simulink model "block_manipulator"  (R2022b)
settings: Solver=ode15s  StartTime=0.0  StopTime=100  FixedStep=0.1  MaxStep=0.01  RelTol=1e-3
values from neighbouring files (symbols this model uses):
  endx = 2    [EnvironmentData.mat]    (also in Practice data.mat = 15)
  endy = 8    [EnvironmentData.mat]    (also in Practice data.mat = 14)
  floorl = 20    [EnvironmentData.mat]    (also in GUIWithNavigation.m; Practice data.mat; RunModel.m)
  floorw = 20    [EnvironmentData.mat]    (also in GUIWithNavigation.m; Practice data.mat; RunModel.m)
  startx = 2    [EnvironmentData.mat]    (also in Practice data.mat)
  starty = 5    [EnvironmentData.mat]    (also in Practice data.mat = 2)
  tar1Len = 3    [EnvironmentData.mat]    (also in GUIWithNavigation.m = length(target1); Practice data.mat = 13; RunModel.m = length(target1))
  target = [2 2.0338184971 1.6 1.6 3.01984057374 1.90928224166 1.77767907717 1.7 5 3.2795509411 2 2 ... (16 elements, 8x2)]    [EnvironmentData.mat]    (also in GUIWithNavigation.m = cat(1,target1,target2); Practice data.mat = [2 3.44057581018 5.07942513831 5.42542290116 7.21306818311 8; RunModel.m = cat(1,target1,target2))
  target1 = [pthObj.States(:,1),pthObj.States(:,2)]    [GUIWithNavigation.m]    (also in RunModel.m)
  target2 = [pthObj.States(:,1),pthObj.States(:,2)]    [GUIWithNavigation.m]    (also in RunModel.m)
undefined symbols (not defined in the file or in its folder): closeFingers, grabObjectAngles, grabObjectAngles2, holdFingers, homeAngles, inverseKinematicWeights, openFingers, readyAngles, X, Y, Z
libraries: sm_lib x199, nesl_utility x57, fl_lib x11, fl_ps_legacy_lib x9, slpidlib x6, robotmaniplib x4
(part 6 of 6)

== system block_manipulator/Manipulator1/j2s6s300_link_finger_3 ==
  Inertia : sm_lib/Body Elements/Inertia  InertiaType=Custom  Mass=0.01  MassUnits=kg  CenterOfMass=[0, 0, 0]  CenterOfMassUnits=m  MomentsOfInertia=[7.8999684e-07, 7.8999684e-07, 8e-08]  MomentsOfInertiaUnits=kg*m^2  ProductsOfInertia=[0, 0, 0]  ProductsOfInertiaUnits=kg*m^2  GraphicType=None  MarkerShape=Inertia  MarkerSize=20  GraphicVisPropType=SimpleVisualProperties  GraphicDiffuseColor=[0.5 0.5 0.5]  GraphicSpecularColor=[0.5 0.5 0.5 1.0]  GraphicAmbientColor=[0.15 0.15 0.15 1.0]  GraphicEmissiveColor=[0.0 0.0 0.0 1.0]  GraphicShininess=75  GraphicOpacity=1.0
  InertiaOriginTransform : sm_lib/Frames and Transforms/Rigid Transform  TranslationMethod=Cartesian  TranslationStandardOffset=0  TranslationLengthUnit=m  TranslationStandardAxis=+Z  TranslationCartesianOffset=[0.022, 0, 0]  TranslationROffset=0  TranslationROffsetUnits=m  TranslationZOffset=0  TranslationZOffsetUnits=m  TranslationThetaOffset=0  TranslationThetaOffsetUnits=deg  RotationMethod=RotationSequence  RotationAngleUnits=deg  RotationStandardAxis=+Z  RotationAngle=0.0  RotationArbitraryAxis=[0 0 1]  FollAlignAxisA=+X  BaseAlignAxisA=+Y  FollAlignAxisB=+Y  BaseAlignAxisB=+Z  RotationSequenceAxes=BaseAxes  RotationSequence=XYZ  RotationSequenceAngles=[0, 0, 0]  RotationSequenceAnglesUnits=rad  RotationMatrix=[1 0 0; 0 1 0; 0 0 1]  Quaternion=[1 0 0 0]
  ReferenceFrame : sm_lib/Frames and Transforms/Reference Frame
  Spatial Contact Force : sm_lib/Forces and Torques/Spatial Contact Force  Commented=on  SenseContactBaseRotation=off  SenseContactBaseTranslation=off  CoefficientOfDynamicFriction=0.3  CoefficientOfStaticFriction=0.5  NormalDamping=1e3  NormalDampingUnits=N/(m/s)  SenseContactSignal=off  NormalStiffness=1e6  NormalStiffnessUnits=N/m  FrictionalCriticalVelocity=1e-3  FrictionalCriticalVelocityUnits=m/s  ZeroCrossDetectContactStartAndEnd=off  SenseContactFollowerRotation=off  SenseContactFollowerTranslation=off  FrictionType=SmoothStickSlip  SenseFrictionalForceMagnitude=off  SenseNormalForceMagnitude=off  NormalForceType=SmoothSpringDamper  SenseNormalVelocity=off  SenseSeparationDistance=off  SenseTangentialVelocity=off  NormalTransitionRegionWidth=1e-4  NormalTransitionRegionWidthUnits=m
  Visual : sm_lib/Body Elements/File Solid  ExtGeomFileName=J2N6S300_finger_proximal.STL  UnitType=Custom  ExtGeomFileUnits=m  StepReaderType=HEX  ExportConvexHullGeometry=on  InertiaType=Custom  Mass=0  MassUnits=kg  CenterOfMass=[0, 0, 0]  CenterOfMassUnits=m  MomentsOfInertia=[0, 0, 0]  MomentsOfInertiaUnits=kg*m^2  ProductsOfInertia=[0, 0, 0]  ProductsOfInertiaUnits=kg*m^2  BasedOnType=DensityFromFile  Density=1000  DensityUnits=kg/m^3  DoExposeReferenceFrame=on  SerializedFrames=<Frames/>  GraphicType=FromGeometry  MarkerShape=Sphere  MarkerSize=10  GraphicVisPropType=SimpleVisualProperties  GraphicDiffuseColor=[0.7254901, 0.490196, 0.062745]  GraphicSpecularColor=[0.5 0.5 0.5 1.0]  GraphicAmbientColor=[0.15 0.15 0.15 1.0]  GraphicEmissiveColor=[0.0 0.0 0.0 1.0]  GraphicShininess=75  GraphicOpacity=1
  VisualOriginTransform : sm_lib/Frames and Transforms/Rigid Transform  TranslationMethod=Cartesian  TranslationStandardOffset=0  TranslationLengthUnit=m  TranslationStandardAxis=+Z  TranslationCartesianOffset=[0, 0, 0]  TranslationROffset=0  TranslationROffsetUnits=m  TranslationZOffset=0  TranslationZOffsetUnits=m  TranslationThetaOffset=0  TranslationThetaOffsetUnits=deg  RotationMethod=RotationSequence  RotationAngleUnits=deg  RotationStandardAxis=+Z  RotationAngle=0.0  RotationArbitraryAxis=[0 0 1]  FollAlignAxisA=+X  BaseAlignAxisA=+Y  FollAlignAxisB=+Y  BaseAlignAxisB=+Z  RotationSequenceAxes=BaseAxes  RotationSequence=XYZ  RotationSequenceAngles=[0, 0, 0]  RotationSequenceAnglesUnits=rad  RotationMatrix=[1 0 0; 0 1 0; 0 0 1]  Quaternion=[1 0 0 0]
  j2s6s300_joint_finger_3_AxisInvTransform : sm_lib/Frames and Transforms/Rigid Transform  TranslationMethod=Cartesian  TranslationStandardOffset=0  TranslationLengthUnit=m  TranslationStandardAxis=+Z  TranslationCartesianOffset=[0, 0, 0]  TranslationROffset=0  TranslationROffsetUnits=m  TranslationZOffset=0  TranslationZOffsetUnits=m  TranslationThetaOffset=0  TranslationThetaOffsetUnits=deg  RotationMethod=ArbitraryAxis  RotationAngleUnits=rad  RotationStandardAxis=+Z  RotationAngle=0  RotationArbitraryAxis=[1, 0, 0]  FollAlignAxisA=+X  BaseAlignAxisA=+Y  FollAlignAxisB=+Y  BaseAlignAxisB=+Z  RotationSequenceAxes=FollowerAxes  RotationSequence=XYX  RotationSequenceAngles=[0 0 0]  RotationSequenceAnglesUnits=deg  RotationMatrix=[1 0 0; 0 1 0; 0 0 1]  Quaternion=[1 0 0 0]
  j2s6s300_joint_finger_tip_3_OriginTransform : sm_lib/Frames and Transforms/Rigid Transform  TranslationMethod=Cartesian  TranslationStandardOffset=0  TranslationLengthUnit=m  TranslationStandardAxis=+Z  TranslationCartesianOffset=[0.044, -0.003, 0]  TranslationROffset=0  TranslationROffsetUnits=m  TranslationZOffset=0  TranslationZOffsetUnits=m  TranslationThetaOffset=0  TranslationThetaOffsetUnits=deg  RotationMethod=RotationSequence  RotationAngleUnits=deg  RotationStandardAxis=+Z  RotationAngle=0.0  RotationArbitraryAxis=[0 0 1]  FollAlignAxisA=+X  BaseAlignAxisA=+Y  FollAlignAxisB=+Y  BaseAlignAxisB=+Z  RotationSequenceAxes=BaseAxes  RotationSequence=XYZ  RotationSequenceAngles=[0, 0, 0]  RotationSequenceAnglesUnits=rad  RotationMatrix=[1 0 0; 0 1 0; 0 0 1]  Quaternion=[1 0 0 0]
  F : PMIOPort  Side=Left
  F1 : PMIOPort  Port=2  Side=Right
  Block1 Contact Force : PMIOPort  Port=3  Side=Right
  connections:
  Inertia/RConn1 -- InertiaOriginTransform/RConn1
  InertiaOriginTransform/LConn1 -- j2s6s300_joint_finger_3_AxisInvTransform/LConn1 -- j2s6s300_joint_finger_tip_3_OriginTransform/LConn1 -- VisualOriginTransform/LConn1 -- ReferenceFrame/RConn1
  Visual/RConn1 -- VisualOriginTransform/RConn1
  j2s6s300_joint_finger_3_AxisInvTransform/RConn1 -- F/RConn1
  j2s6s300_joint_finger_tip_3_OriginTransform/RConn1 -- F1/RConn1
  Spatial Contact Force/RConn1 -- Block1 Contact Force/RConn1
  Spatial Contact Force/LConn1 -- Visual/LConn1

== system block_manipulator/Manipulator1/j2s6s300_link_finger_tip_1 ==
  Inertia : sm_lib/Body Elements/Inertia  InertiaType=Custom  Mass=0.01  MassUnits=kg  CenterOfMass=[0, 0, 0]  CenterOfMassUnits=m  MomentsOfInertia=[7.8999684e-07, 7.8999684e-07, 8e-08]  MomentsOfInertiaUnits=kg*m^2  ProductsOfInertia=[0, 0, 0]  ProductsOfInertiaUnits=kg*m^2  GraphicType=None  MarkerShape=Inertia  MarkerSize=20  GraphicVisPropType=SimpleVisualProperties  GraphicDiffuseColor=[0.5 0.5 0.5]  GraphicSpecularColor=[0.5 0.5 0.5 1.0]  GraphicAmbientColor=[0.15 0.15 0.15 1.0]  GraphicEmissiveColor=[0.0 0.0 0.0 1.0]  GraphicShininess=75  GraphicOpacity=1.0
  InertiaOriginTransform : sm_lib/Frames and Transforms/Rigid Transform  TranslationMethod=Cartesian  TranslationStandardOffset=0  TranslationLengthUnit=m  TranslationStandardAxis=+Z  TranslationCartesianOffset=[0.022, 0, 0]  TranslationROffset=0  TranslationROffsetUnits=m  TranslationZOffset=0  TranslationZOffsetUnits=m  TranslationThetaOffset=0  TranslationThetaOffsetUnits=deg  RotationMethod=RotationSequence  RotationAngleUnits=deg  RotationStandardAxis=+Z  RotationAngle=0.0  RotationArbitraryAxis=[0 0 1]  FollAlignAxisA=+X  BaseAlignAxisA=+Y  FollAlignAxisB=+Y  BaseAlignAxisB=+Z  RotationSequenceAxes=BaseAxes  RotationSequence=XYZ  RotationSequenceAngles=[0, 0, 0]  RotationSequenceAnglesUnits=rad  RotationMatrix=[1 0 0; 0 1 0; 0 0 1]  Quaternion=[1 0 0 0]
  ReferenceFrame : sm_lib/Frames and Transforms/Reference Frame
  Spatial Contact Force : sm_lib/Forces and Torques/Spatial Contact Force  Commented=on  SenseContactBaseRotation=off  SenseContactBaseTranslation=off  CoefficientOfDynamicFriction=0.9  CoefficientOfStaticFriction=0.9  NormalDamping=1e3  NormalDampingUnits=N/(m/s)  SenseContactSignal=off  NormalStiffness=1e6  NormalStiffnessUnits=N/m  FrictionalCriticalVelocity=1e-3  FrictionalCriticalVelocityUnits=m/s  ZeroCrossDetectContactStartAndEnd=off  SenseContactFollowerRotation=off  SenseContactFollowerTranslation=off  FrictionType=SmoothStickSlip  SenseFrictionalForceMagnitude=off  SenseNormalForceMagnitude=on  NormalForceType=SmoothSpringDamper  SenseNormalVelocity=off  SenseSeparationDistance=off  SenseTangentialVelocity=off  NormalTransitionRegionWidth=1e-4  NormalTransitionRegionWidthUnits=m
  Visual : sm_lib/Body Elements/File Solid  ExtGeomFileName=J2N6S300_finger_distal.STL  UnitType=Custom  ExtGeomFileUnits=m  StepReaderType=HEX  ExportConvexHullGeometry=on  InertiaType=Custom  Mass=0  MassUnits=kg  CenterOfMass=[0, 0, 0]  CenterOfMassUnits=m  MomentsOfInertia=[0, 0, 0]  MomentsOfInertiaUnits=kg*m^2  ProductsOfInertia=[0, 0, 0]  ProductsOfInertiaUnits=kg*m^2  BasedOnType=DensityFromFile  Density=1000  DensityUnits=kg/m^3  DoExposeReferenceFrame=on  SerializedFrames=<Frames/>  GraphicType=FromGeometry  MarkerShape=Sphere  MarkerSize=10  GraphicVisPropType=SimpleVisualProperties  GraphicDiffuseColor=[0.4156862, 0.0470588, 0.0431372]  GraphicSpecularColor=[0.5 0.5 0.5 1.0]  GraphicAmbientColor=[0.15 0.15 0.15 1.0]  GraphicEmissiveColor=[0.0 0.0 0.0 1.0]  GraphicShininess=75  GraphicOpacity=1
  VisualOriginTransform : sm_lib/Frames and Transforms/Rigid Transform  TranslationMethod=Cartesian  TranslationStandardOffset=0  TranslationLengthUnit=m  TranslationStandardAxis=+Z  TranslationCartesianOffset=[0, 0, 0]  TranslationROffset=0  TranslationROffsetUnits=m  TranslationZOffset=0  TranslationZOffsetUnits=m  TranslationThetaOffset=0  TranslationThetaOffsetUnits=deg  RotationMethod=RotationSequence  RotationAngleUnits=deg  RotationStandardAxis=+Z  RotationAngle=0.0  RotationArbitraryAxis=[0 0 1]  FollAlignAxisA=+X  BaseAlignAxisA=+Y  FollAlignAxisB=+Y  BaseAlignAxisB=+Z  RotationSequenceAxes=BaseAxes  RotationSequence=XYZ  RotationSequenceAngles=[0, 0, 0]  RotationSequenceAnglesUnits=rad  RotationMatrix=[1 0 0; 0 1 0; 0 0 1]  Quaternion=[1 0 0 0]
  F : PMIOPort  Side=Left
  Block1 Contact Force : PMIOPort  Port=2  Side=Right
  F1 : PMIOPort  Port=3  Side=Left
  connections:
  Inertia/RConn1 -- InertiaOriginTransform/RConn1
  InertiaOriginTransform/LConn1 -- ReferenceFrame/RConn1 -- F/RConn1 -- VisualOriginTransform/LConn1
  Visual/RConn1 -- VisualOriginTransform/RConn1
  Visual/LConn1 -- Spatial Contact Force/LConn1
  Spatial Contact Force/RConn1 -- Block1 Contact Force/RConn1
  F1/RConn1 -- Spatial Contact Force/RConn2

== system block_manipulator/Manipulator1/j2s6s300_link_finger_tip_2 ==
  Inertia : sm_lib/Body Elements/Inertia  InertiaType=Custom  Mass=0.01  MassUnits=kg  CenterOfMass=[0, 0, 0]  CenterOfMassUnits=m  MomentsOfInertia=[7.8999684e-07, 7.8999684e-07, 8e-08]  MomentsOfInertiaUnits=kg*m^2  ProductsOfInertia=[0, 0, 0]  ProductsOfInertiaUnits=kg*m^2  GraphicType=None  MarkerShape=Inertia  MarkerSize=20  GraphicVisPropType=SimpleVisualProperties  GraphicDiffuseColor=[0.5 0.5 0.5]  GraphicSpecularColor=[0.5 0.5 0.5 1.0]  GraphicAmbientColor=[0.15 0.15 0.15 1.0]  GraphicEmissiveColor=[0.0 0.0 0.0 1.0]  GraphicShininess=75  GraphicOpacity=1.0
  InertiaOriginTransform : sm_lib/Frames and Transforms/Rigid Transform  TranslationMethod=Cartesian  TranslationStandardOffset=0  TranslationLengthUnit=m  TranslationStandardAxis=+Z  TranslationCartesianOffset=[0.022, 0, 0]  TranslationROffset=0  TranslationROffsetUnits=m  TranslationZOffset=0  TranslationZOffsetUnits=m  TranslationThetaOffset=0  TranslationThetaOffsetUnits=deg  RotationMethod=RotationSequence  RotationAngleUnits=deg  RotationStandardAxis=+Z  RotationAngle=0.0  RotationArbitraryAxis=[0 0 1]  FollAlignAxisA=+X  BaseAlignAxisA=+Y  FollAlignAxisB=+Y  BaseAlignAxisB=+Z  RotationSequenceAxes=BaseAxes  RotationSequence=XYZ  RotationSequenceAngles=[0, 0, 0]  RotationSequenceAnglesUnits=rad  RotationMatrix=[1 0 0; 0 1 0; 0 0 1]  Quaternion=[1 0 0 0]
  ReferenceFrame : sm_lib/Frames and Transforms/Reference Frame
  Spatial Contact Force : sm_lib/Forces and Torques/Spatial Contact Force  Commented=on  SenseContactBaseRotation=off  SenseContactBaseTranslation=off  CoefficientOfDynamicFriction=0.9  CoefficientOfStaticFriction=0.9  NormalDamping=1e3  NormalDampingUnits=N/(m/s)  SenseContactSignal=off  NormalStiffness=1e6  NormalStiffnessUnits=N/m  FrictionalCriticalVelocity=1e-3  FrictionalCriticalVelocityUnits=m/s  ZeroCrossDetectContactStartAndEnd=off  SenseContactFollowerRotation=off  SenseContactFollowerTranslation=off  FrictionType=SmoothStickSlip  SenseFrictionalForceMagnitude=off  SenseNormalForceMagnitude=on  NormalForceType=SmoothSpringDamper  SenseNormalVelocity=off  SenseSeparationDistance=off  SenseTangentialVelocity=off  NormalTransitionRegionWidth=1e-4  NormalTransitionRegionWidthUnits=m
  Visual : sm_lib/Body Elements/File Solid  ExtGeomFileName=J2N6S300_finger_distal.STL  UnitType=Custom  ExtGeomFileUnits=m  StepReaderType=HEX  ExportConvexHullGeometry=on  InertiaType=Custom  Mass=0  MassUnits=kg  CenterOfMass=[0, 0, 0]  CenterOfMassUnits=m  MomentsOfInertia=[0, 0, 0]  MomentsOfInertiaUnits=kg*m^2  ProductsOfInertia=[0, 0, 0]  ProductsOfInertiaUnits=kg*m^2  BasedOnType=DensityFromFile  Density=1000  DensityUnits=kg/m^3  DoExposeReferenceFrame=on  SerializedFrames=<Frames/>  GraphicType=FromGeometry  MarkerShape=Sphere  MarkerSize=10  GraphicVisPropType=SimpleVisualProperties  GraphicDiffuseColor=[0.4156862, 0.0470588, 0.0431372]  GraphicSpecularColor=[0.5 0.5 0.5 1.0]  GraphicAmbientColor=[0.15 0.15 0.15 1.0]  GraphicEmissiveColor=[0.0 0.0 0.0 1.0]  GraphicShininess=75  GraphicOpacity=1
  VisualOriginTransform : sm_lib/Frames and Transforms/Rigid Transform  TranslationMethod=Cartesian  TranslationStandardOffset=0  TranslationLengthUnit=m  TranslationStandardAxis=+Z  TranslationCartesianOffset=[0, 0, 0]  TranslationROffset=0  TranslationROffsetUnits=m  TranslationZOffset=0  TranslationZOffsetUnits=m  TranslationThetaOffset=0  TranslationThetaOffsetUnits=deg  RotationMethod=RotationSequence  RotationAngleUnits=deg  RotationStandardAxis=+Z  RotationAngle=0.0  RotationArbitraryAxis=[0 0 1]  FollAlignAxisA=+X  BaseAlignAxisA=+Y  FollAlignAxisB=+Y  BaseAlignAxisB=+Z  RotationSequenceAxes=BaseAxes  RotationSequence=XYZ  RotationSequenceAngles=[0, 0, 0]  RotationSequenceAnglesUnits=rad  RotationMatrix=[1 0 0; 0 1 0; 0 0 1]  Quaternion=[1 0 0 0]
  F : PMIOPort  Side=Left
  Block1 Contact Force : PMIOPort  Port=2  Side=Right
  F1 : PMIOPort  Port=3  Side=Left
  connections:
  Inertia/RConn1 -- InertiaOriginTransform/RConn1
  InertiaOriginTransform/LConn1 -- ReferenceFrame/RConn1 -- F/RConn1 -- VisualOriginTransform/LConn1
  Visual/RConn1 -- VisualOriginTransform/RConn1
  Visual/LConn1 -- Spatial Contact Force/LConn1
  Block1 Contact Force/RConn1 -- Spatial Contact Force/RConn1
  Spatial Contact Force/RConn2 -- F1/RConn1

== system block_manipulator/Manipulator1/j2s6s300_link_finger_tip_3 ==
  Inertia : sm_lib/Body Elements/Inertia  InertiaType=Custom  Mass=0.01  MassUnits=kg  CenterOfMass=[0, 0, 0]  CenterOfMassUnits=m  MomentsOfInertia=[7.8999684e-07, 7.8999684e-07, 8e-08]  MomentsOfInertiaUnits=kg*m^2  ProductsOfInertia=[0, 0, 0]  ProductsOfInertiaUnits=kg*m^2  GraphicType=None  MarkerShape=Inertia  MarkerSize=20  GraphicVisPropType=SimpleVisualProperties  GraphicDiffuseColor=[0.5 0.5 0.5]  GraphicSpecularColor=[0.5 0.5 0.5 1.0]  GraphicAmbientColor=[0.15 0.15 0.15 1.0]  GraphicEmissiveColor=[0.0 0.0 0.0 1.0]  GraphicShininess=75  GraphicOpacity=1.0
  InertiaOriginTransform : sm_lib/Frames and Transforms/Rigid Transform  TranslationMethod=Cartesian  TranslationStandardOffset=0  TranslationLengthUnit=m  TranslationStandardAxis=+Z  TranslationCartesianOffset=[0.022, 0, 0]  TranslationROffset=0  TranslationROffsetUnits=m  TranslationZOffset=0  TranslationZOffsetUnits=m  TranslationThetaOffset=0  TranslationThetaOffsetUnits=deg  RotationMethod=RotationSequence  RotationAngleUnits=deg  RotationStandardAxis=+Z  RotationAngle=0.0  RotationArbitraryAxis=[0 0 1]  FollAlignAxisA=+X  BaseAlignAxisA=+Y  FollAlignAxisB=+Y  BaseAlignAxisB=+Z  RotationSequenceAxes=BaseAxes  RotationSequence=XYZ  RotationSequenceAngles=[0, 0, 0]  RotationSequenceAnglesUnits=rad  RotationMatrix=[1 0 0; 0 1 0; 0 0 1]  Quaternion=[1 0 0 0]
  ReferenceFrame : sm_lib/Frames and Transforms/Reference Frame
  Spatial Contact Force : sm_lib/Forces and Torques/Spatial Contact Force  Commented=on  SenseContactBaseRotation=off  SenseContactBaseTranslation=off  CoefficientOfDynamicFriction=0.9  CoefficientOfStaticFriction=0.9  NormalDamping=1e3  NormalDampingUnits=N/(m/s)  SenseContactSignal=off  NormalStiffness=1e6  NormalStiffnessUnits=N/m  FrictionalCriticalVelocity=1e-3  FrictionalCriticalVelocityUnits=m/s  ZeroCrossDetectContactStartAndEnd=off  SenseContactFollowerRotation=off  SenseContactFollowerTranslation=off  FrictionType=SmoothStickSlip  SenseFrictionalForceMagnitude=off  SenseNormalForceMagnitude=on  NormalForceType=SmoothSpringDamper  SenseNormalVelocity=off  SenseSeparationDistance=off  SenseTangentialVelocity=off  NormalTransitionRegionWidth=1e-4  NormalTransitionRegionWidthUnits=m
  Visual : sm_lib/Body Elements/File Solid  ExtGeomFileName=J2N6S300_finger_distal.STL  UnitType=Custom  ExtGeomFileUnits=m  StepReaderType=HEX  ExportConvexHullGeometry=on  InertiaType=Custom  Mass=0  MassUnits=kg  CenterOfMass=[0, 0, 0]  CenterOfMassUnits=m  MomentsOfInertia=[0, 0, 0]  MomentsOfInertiaUnits=kg*m^2  ProductsOfInertia=[0, 0, 0]  ProductsOfInertiaUnits=kg*m^2  BasedOnType=DensityFromFile  Density=1000  DensityUnits=kg/m^3  DoExposeReferenceFrame=on  SerializedFrames=<Frames/>  GraphicType=FromGeometry  MarkerShape=Sphere  MarkerSize=10  GraphicVisPropType=SimpleVisualProperties  GraphicDiffuseColor=[0.4156862, 0.0470588, 0.0431372]  GraphicSpecularColor=[0.5 0.5 0.5 1.0]  GraphicAmbientColor=[0.15 0.15 0.15 1.0]  GraphicEmissiveColor=[0.0 0.0 0.0 1.0]  GraphicShininess=75  GraphicOpacity=1
  VisualOriginTransform : sm_lib/Frames and Transforms/Rigid Transform  TranslationMethod=Cartesian  TranslationStandardOffset=0  TranslationLengthUnit=m  TranslationStandardAxis=+Z  TranslationCartesianOffset=[0, 0, 0]  TranslationROffset=0  TranslationROffsetUnits=m  TranslationZOffset=0  TranslationZOffsetUnits=m  TranslationThetaOffset=0  TranslationThetaOffsetUnits=deg  RotationMethod=RotationSequence  RotationAngleUnits=deg  RotationStandardAxis=+Z  RotationAngle=0.0  RotationArbitraryAxis=[0 0 1]  FollAlignAxisA=+X  BaseAlignAxisA=+Y  FollAlignAxisB=+Y  BaseAlignAxisB=+Z  RotationSequenceAxes=BaseAxes  RotationSequence=XYZ  RotationSequenceAngles=[0, 0, 0]  RotationSequenceAnglesUnits=rad  RotationMatrix=[1 0 0; 0 1 0; 0 0 1]  Quaternion=[1 0 0 0]
  F : PMIOPort  Side=Left
  Block1 Contact Force : PMIOPort  Port=2  Side=Right
  F1 : PMIOPort  Port=3  Side=Left
  connections:
  Inertia/RConn1 -- InertiaOriginTransform/RConn1
  InertiaOriginTransform/LConn1 -- ReferenceFrame/RConn1 -- F/RConn1 -- VisualOriginTransform/LConn1
  Visual/RConn1 -- VisualOriginTransform/RConn1
  Visual/LConn1 -- Spatial Contact Force/LConn1
  Block1 Contact Force/RConn1 -- Spatial Contact Force/RConn1
  F1/RConn1 -- Spatial Contact Force/RConn2

== system block_manipulator/Controller/Path follower/If Action Subsystem ==
  In1 : Inport
  Action Port : ActionPort  ActionPortLabel=if(u1 <= 0)
  Out1 : Outport
  wires:
  In1/1 -> Out1/1

== system block_manipulator/Controller/Path follower/If Action Subsystem1 ==
  In1 : Inport
  Action Port : ActionPort  ActionPortLabel=else
  Out1 : Outport
  wires:
  In1/1 -> Out1/1

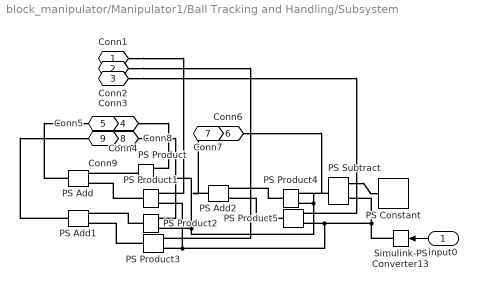
== system block_manipulator/Manipulator1/Ball Tracking and Handling/Subsystem ==
  input0 : Inport
  PS Add : fl_lib/Physical Signals/Functions/PS Add
  PS Add1 : fl_lib/Physical Signals/Functions/PS Add
  PS Add2 : fl_lib/Physical Signals/Functions/PS Add
  PS Constant : fl_lib/Physical Signals/Sources/PS Constant  constant=1
  PS Product{,1..5} (6 alike) : fl_ps_legacy_lib/Legacy Physical Signals/Functions/PS Product
  PS Subtract : fl_lib/Physical Signals/Functions/PS Subtract
  Simulink-PS Converter13 : nesl_utility/Simulink-PS Converter  PhysicalDomain=network_engine_domain  SubClassName=ps_input  LeftPortType=input  RightPortType=output  PseudoPeriodic=off  Frequencies=[]  NoiseDistribution=none  NoiseParameters=[]  Unit=1  AffineConversion=off  FilteringAndDerivatives=provide  SimscapeFilterOrder=1  InputFilterTimeConstant=0.001  UdotUserProvided=0
  Conn1 : PMIOPort  Side=Left
  Conn2 : PMIOPort  Port=2  Side=Left
  Conn3 : PMIOPort  Port=3  Side=Left
  Conn4 : PMIOPort  Port=4  Side=Right
  Conn5 : PMIOPort  Port=5  Side=Left
  Conn6 : PMIOPort  Port=6  Side=Right
  Conn7 : PMIOPort  Port=7  Side=Left
  Conn8 : PMIOPort  Port=8  Side=Right
  Conn9 : PMIOPort  Port=9  Side=Left
  wires:
  input0/1 -> Simulink-PS Converter13/1
  connections:
  PS Product3/RConn1 -- PS Add1/LConn2
  PS Subtract/RConn1 -- PS Product/LConn1 -- PS Product2/LConn1 -- PS Product4/LConn1
  PS Product/RConn1 -- PS Add/LConn1
  PS Product4/RConn1 -- PS Add2/LConn1
  Conn2/RConn1 -- PS Product3/LConn2
  PS Add1/RConn1 -- Conn8/RConn1
  PS Product2/RConn1 -- PS Add1/LConn1
  PS Product5/RConn1 -- PS Add2/LConn2
  PS Subtract/LConn1 -- PS Constant/RConn1
  Simulink-PS Converter13/RConn1 -- PS Product1/LConn1 -- PS Product3/LConn1 -- PS Product5/LConn1 -- PS Subtract/LConn2
  PS Product1/RConn1 -- PS Add/LConn2
  Conn7/RConn1 -- PS Product4/LConn2
  Conn5/RConn1 -- PS Product/LConn2
  Conn9/RConn1 -- PS Product2/LConn2
  PS Add/RConn1 -- Conn4/RConn1
  Conn3/RConn1 -- PS Product5/LConn2
  Conn1/RConn1 -- PS Product1/LConn2
  PS Add2/RConn1 -- Conn6/RConn1

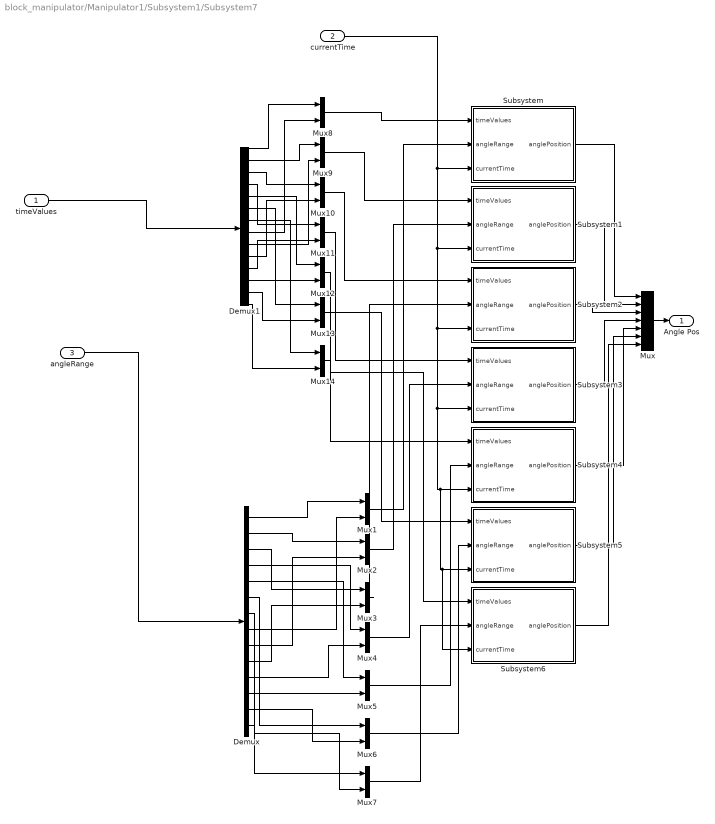
== system block_manipulator/Manipulator1/Subsystem1/Subsystem7 ==
  timeValues : Inport  PortDimensions=[1 14]
  currentTime : Inport  Port=2
  angleRange : Inport  Port=3
  Demux : Demux  Outputs=14
  Demux1 : Demux  Outputs=14
  Mux : Mux  Inputs=7
  Mux{1..14} (14 alike) : Mux  Inputs=2
  Subsystem : Subsystem
  Subsystem1 : Subsystem
  Subsystem2 : Subsystem
  Subsystem3 : Subsystem
  Subsystem4 : Subsystem
  Subsystem5 : Subsystem
  Subsystem6 : Subsystem
  Angle Pos : Outport
  wires:
  Subsystem3/1(anglePosition) -> Mux/4
  currentTime/1 -> Subsystem6/3(currentTime), Subsystem5/3(currentTime), Subsystem4/3(currentTime), Subsystem3/3(currentTime), Subsystem2/3(currentTime), Subsystem1/3(currentTime), Subsystem/3(currentTime)
  Subsystem2/1(anglePosition) -> Mux/3
  Subsystem/1(anglePosition) -> Mux/1
  Subsystem4/1(anglePosition) -> Mux/5
  angleRange/1 -> Demux/1
  Subsystem1/1(anglePosition) -> Mux/2
  Subsystem5/1(anglePosition) -> Mux/6
  Subsystem6/1(anglePosition) -> Mux/7
  Mux/1 -> Angle Pos/1
  Demux/1 -> Mux1/1
  Demux/8 -> Mux1/2
  Demux/2 -> Mux2/1
  Demux/9 -> Mux2/2
  Demux/3 -> Mux3/1
  Demux/10 -> Mux3/2
  Demux/4 -> Mux4/1
  Demux/11 -> Mux4/2
  Demux/5 -> Mux5/1
  Demux/12 -> Mux5/2
  Demux/6 -> Mux6/1
  Demux/13 -> Mux6/2
  Demux/7 -> Mux7/1
  Demux/14 -> Mux7/2
  Mux1/1 -> Subsystem/2(angleRange)
  Mux2/1 -> Subsystem1/2(angleRange)
  Mux3/1 -> Subsystem2/2(angleRange)
  Mux4/1 -> Subsystem3/2(angleRange)
  Mux5/1 -> Subsystem4/2(angleRange)
  Mux6/1 -> Subsystem5/2(angleRange)
  Mux7/1 -> Subsystem6/2(angleRange)
  Demux1/1 -> Mux8/1
  Demux1/2 -> Mux9/1
  Demux1/8 -> Mux8/2
  Demux1/3 -> Mux10/1
  Demux1/9 -> Mux9/2
  Demux1/10 -> Mux10/2
  Demux1/4 -> Mux11/1
  Demux1/11 -> Mux11/2
  Demux1/5 -> Mux12/1
  Demux1/12 -> Mux12/2
  Demux1/6 -> Mux13/1
  Demux1/13 -> Mux13/2
  Demux1/7 -> Mux14/1
  Demux1/14 -> Mux14/2
  Mux8/1 -> Subsystem/1(timeValues)
  Mux9/1 -> Subsystem1/1(timeValues)
  Mux10/1 -> Subsystem2/1(timeValues)
  Mux11/1 -> Subsystem3/1(timeValues)
  Mux12/1 -> Subsystem4/1(timeValues)
  Mux13/1 -> Subsystem5/1(timeValues)
  Mux14/1 -> Subsystem6/1(timeValues)
  timeValues/1 -> Demux1/1

== system block_manipulator/Manipulator1/inverseKinematics/If Action Subsystem ==
  T : Inport
  Action Port : ActionPort  ActionPortLabel=if(u1==1&u2==0)
  Constant7 : Constant  Value=inverseKinematicWeights
  Constant8 : Constant  Value=homeAngles
  Inverse Kinematics : robotmaniplib/Inverse Kinematics  RigidBodyTree=manipulatorModel  EndEffector=grabPositionBody  ShowInfo=off  SolverName=BFGS Gradient Projection  EnforceJointLimits=on  MaxIterations=1500  MaxTime=10  GradientTolerance=1e-7  SolutionTolerance=1e-6  StepTolerance=1e-14  ErrorChangeTolerance=1e-12  UseErrorDamping=on  DampingBias=0.0025  SimulateUsing=Interpreted execution
  objectPosition : Outport
  wires:
  Constant8/1 -> Inverse Kinematics/3
  Constant7/1 -> Inverse Kinematics/2
  T/1 -> Inverse Kinematics/1
  Inverse Kinematics/1 -> objectPosition/1

== system block_manipulator/Manipulator1/inverseKinematics/If Action Subsystem1 ==
  Action Port : ActionPort  ActionPortLabel=else

== system block_manipulator/Manipulator1/inverseKinematics/If Action Subsystem2 ==
  T : Inport
  Action Port : ActionPort  ActionPortLabel=if(u1==1&u2==0)
  Constant7 : Constant  Value=inverseKinematicWeights
  Constant8 : Constant  Value=homeAngles
  Inverse Kinematics : robotmaniplib/Inverse Kinematics  RigidBodyTree=manipulatorModel  EndEffector=grabPositionBody  ShowInfo=off  SolverName=BFGS Gradient Projection  EnforceJointLimits=on  MaxIterations=1500  MaxTime=10  GradientTolerance=1e-7  SolutionTolerance=1e-6  StepTolerance=1e-14  ErrorChangeTolerance=1e-12  UseErrorDamping=on  DampingBias=0.0025  SimulateUsing=Interpreted execution
  objectPosition : Outport
  wires:
  Constant8/1 -> Inverse Kinematics/3
  Constant7/1 -> Inverse Kinematics/2
  T/1 -> Inverse Kinematics/1
  Inverse Kinematics/1 -> objectPosition/1

== system block_manipulator/Manipulator1/inverseKinematics/If Action Subsystem3 ==
  Action Port : ActionPort  ActionPortLabel=else

== system block_manipulator/Manipulator1/inverseKinematics1/If Action Subsystem ==
  T : Inport
  Action Port : ActionPort
  Constant7 : Constant  Value=inverseKinematicWeights
  Constant8 : Constant  Value=homeAngles
  Inverse Kinematics : robotmaniplib/Inverse Kinematics  RigidBodyTree=manipulatorModel  EndEffector=grabPositionBody  ShowInfo=off  SolverName=BFGS Gradient Projection  EnforceJointLimits=on  MaxIterations=1500  MaxTime=10  GradientTolerance=1e-7  SolutionTolerance=1e-6  StepTolerance=1e-14  ErrorChangeTolerance=1e-12  UseErrorDamping=on  DampingBias=0.0025  SimulateUsing=Interpreted execution
  objectPosition : Outport
  wires:
  Constant8/1 -> Inverse Kinematics/3
  Constant7/1 -> Inverse Kinematics/2
  T/1 -> Inverse Kinematics/1
  Inverse Kinematics/1 -> objectPosition/1

== system block_manipulator/Manipulator1/inverseKinematics1/If Action Subsystem1 ==
  Action Port : ActionPort

== system block_manipulator/Manipulator1/inverseKinematics1/If Action Subsystem2 ==
  T : Inport
  Action Port : ActionPort
  Constant7 : Constant  Value=inverseKinematicWeights
  Constant8 : Constant  Value=homeAngles
  Inverse Kinematics : robotmaniplib/Inverse Kinematics  RigidBodyTree=manipulatorModel  EndEffector=grabPositionBody  ShowInfo=off  SolverName=BFGS Gradient Projection  EnforceJointLimits=on  MaxIterations=1500  MaxTime=10  GradientTolerance=1e-7  SolutionTolerance=1e-6  StepTolerance=1e-14  ErrorChangeTolerance=1e-12  UseErrorDamping=on  DampingBias=0.0025  SimulateUsing=Interpreted execution
  objectPosition : Outport
  wires:
  Constant8/1 -> Inverse Kinematics/3
  Constant7/1 -> Inverse Kinematics/2
  T/1 -> Inverse Kinematics/1
  Inverse Kinematics/1 -> objectPosition/1

== system block_manipulator/Manipulator1/inverseKinematics1/If Action Subsystem3 ==
  Action Port : ActionPort

== system block_manipulator/Manipulator1/Subsystem1/Subsystem7/Subsystem ==
  timeValues : Inport
  angleRange : Inport  Port=2
  currentTime : Inport  Port=3
  1-D Lookup Table : Lookup_n-D  NumberOfTableDimensions=1  BreakpointsForDimension1Source=Input port  BreakpointsForDimension1=[-5:5]  TableSource=Input port  Table=tanh([-5:5])  InternalRulePriority=Speed  RndMeth=Simplest
      settings: InputPortMap=u0,p221,p5
  Display : Display
  anglePosition : Outport
  wires:
  timeValues/1 -> 1-D Lookup Table/3
  1-D Lookup Table/1 -> anglePosition/1
  currentTime/1 -> 1-D Lookup Table/1
  angleRange/1 -> 1-D Lookup Table/2, Display/1

== system block_manipulator/Manipulator1/Subsystem1/Subsystem7/Subsystem1 ==
  timeValues : Inport
  angleRange : Inport  Port=2
  currentTime : Inport  Port=3
  1-D Lookup Table : Lookup_n-D  NumberOfTableDimensions=1  BreakpointsForDimension1Source=Input port  BreakpointsForDimension1=[-5:5]  TableSource=Input port  Table=tanh([-5:5])  InternalRulePriority=Speed  RndMeth=Simplest
      settings: InputPortMap=u0,p221,p5
  anglePosition : Outport
  wires:
  timeValues/1 -> 1-D Lookup Table/3
  1-D Lookup Table/1 -> anglePosition/1
  currentTime/1 -> 1-D Lookup Table/1
  angleRange/1 -> 1-D Lookup Table/2

== system block_manipulator/Manipulator1/Subsystem1/Subsystem7/Subsystem2 ==
  timeValues : Inport
  angleRange : Inport  Port=2
  currentTime : Inport  Port=3
  1-D Lookup Table : Lookup_n-D  NumberOfTableDimensions=1  BreakpointsForDimension1Source=Input port  BreakpointsForDimension1=[-5:5]  TableSource=Input port  Table=tanh([-5:5])  InternalRulePriority=Speed  RndMeth=Simplest
      settings: InputPortMap=u0,p221,p5
  anglePosition : Outport
  wires:
  timeValues/1 -> 1-D Lookup Table/3
  1-D Lookup Table/1 -> anglePosition/1
  currentTime/1 -> 1-D Lookup Table/1
  angleRange/1 -> 1-D Lookup Table/2

== system block_manipulator/Manipulator1/Subsystem1/Subsystem7/Subsystem3 ==
  timeValues : Inport
  angleRange : Inport  Port=2
  currentTime : Inport  Port=3
  1-D Lookup Table : Lookup_n-D  NumberOfTableDimensions=1  BreakpointsForDimension1Source=Input port  BreakpointsForDimension1=[-5:5]  TableSource=Input port  Table=tanh([-5:5])  InternalRulePriority=Speed  RndMeth=Simplest
      settings: InputPortMap=u0,p221,p5
  anglePosition : Outport
  wires:
  timeValues/1 -> 1-D Lookup Table/3
  1-D Lookup Table/1 -> anglePosition/1
  currentTime/1 -> 1-D Lookup Table/1
  angleRange/1 -> 1-D Lookup Table/2

== system block_manipulator/Manipulator1/Subsystem1/Subsystem7/Subsystem4 ==
  timeValues : Inport
  angleRange : Inport  Port=2
  currentTime : Inport  Port=3
  1-D Lookup Table : Lookup_n-D  NumberOfTableDimensions=1  BreakpointsForDimension1Source=Input port  BreakpointsForDimension1=[-5:5]  TableSource=Input port  Table=tanh([-5:5])  InternalRulePriority=Speed  RndMeth=Simplest
      settings: InputPortMap=u0,p221,p5
  anglePosition : Outport
  wires:
  timeValues/1 -> 1-D Lookup Table/3
  1-D Lookup Table/1 -> anglePosition/1
  currentTime/1 -> 1-D Lookup Table/1
  angleRange/1 -> 1-D Lookup Table/2

== system block_manipulator/Manipulator1/Subsystem1/Subsystem7/Subsystem5 ==
  timeValues : Inport
  angleRange : Inport  Port=2
  currentTime : Inport  Port=3
  1-D Lookup Table : Lookup_n-D  NumberOfTableDimensions=1  BreakpointsForDimension1Source=Input port  BreakpointsForDimension1=[-5:5]  TableSource=Input port  Table=tanh([-5:5])  InternalRulePriority=Speed  RndMeth=Simplest
      settings: InputPortMap=u0,p221,p5
  anglePosition : Outport
  wires:
  timeValues/1 -> 1-D Lookup Table/3
  1-D Lookup Table/1 -> anglePosition/1
  currentTime/1 -> 1-D Lookup Table/1
  angleRange/1 -> 1-D Lookup Table/2

== system block_manipulator/Manipulator1/Subsystem1/Subsystem7/Subsystem6 ==
  timeValues : Inport
  angleRange : Inport  Port=2
  currentTime : Inport  Port=3
  1-D Lookup Table : Lookup_n-D  NumberOfTableDimensions=1  BreakpointsForDimension1Source=Input port  BreakpointsForDimension1=[-5:5]  TableSource=Input port  Table=tanh([-5:5])  InternalRulePriority=Speed  RndMeth=Simplest
      settings: InputPortMap=u0,p221,p5
  anglePosition : Outport
  wires:
  timeValues/1 -> 1-D Lookup Table/3
  1-D Lookup Table/1 -> anglePosition/1
  currentTime/1 -> 1-D Lookup Table/1
  angleRange/1 -> 1-D Lookup Table/2

== stateflow chart block_manipulator/Controller/Chart ==
  state PathFollowing
    resetPos=0;
  state ManipulatorTask
    resetPos=1;
  (default) -> PathFollowing
  PathFollowing -> ManipulatorTask : [(pos_index>tar1Len)&&(manipState<5)]
  ManipulatorTask -> PathFollowing : [manipState>=5]
  data: pos_index input; tar1Len input; resetPos output; manipState input

== matlab function block_manipulator/Manipulator1/End Tracking and handling/MATLAB Function1 ==
  data: objectTransform output; x input; y input; z input; aboveObjectTransform output
function [objectTransform,aboveObjectTransform] = fcn(x,y,z)
rotTransform=[1 0 0;0 -1 0;0 0 -1];
F=rotTransform;
xline=F(1,:);
yline=F(2,:);
zline=F(3,:);
objectTransform = [ xline x;yline y;zline z+0.02;0 0 0 1];
aboveObjectTransform = [xline x;yline y;zline z+0.1;0 0 0 1];

== matlab function block_manipulator/Manipulator1/MATLAB Function ==
  settings: updateMethod=DISCRETE
  data: quadrupedInPosition input; errorVals input; contactForces input; state input; y output; readyAngles input; grabObjectAngles2 input; grabObjectAngles input; openFingers input; closeFingers input; holdFingers input; stateOut output; objectPosition input; aboveObjectPosition input; getBallPos output; getEndPos output; ballGot output; endPos input; aboveEndPos input
function [y,stateOut,getBallPos,getEndPos,ballGot] = fcn(quadrupedInPosition,errorVals,contactForces,state,readyAngles,grabObjectAngles2,grabObjectAngles,openFingers,closeFingers,holdFingers,objectPosition,aboveObjectPosition,endPos,aboveEndPos)


if quadrupedInPosition == 1
    state = int16(state);

    switch state
        case 0
            y = [readyAngles;openFingers];
            getBallPos=0;
            getEndPos=0;
            ballGot=0;
        case 1
            getBallPos=0;
            getEndPos=0;
            y = [aboveObjectPosition;openFingers];
            ballGot=0;
        case 2
            getBallPos=0;
            getEndPos=0;
            y = [objectPosition;openFingers];
            ballGot=0;
        case 3
            getBallPos=0;
            getEndPos=0;
            y = [objectPosition;closeFingers];
            ballGot=0;
        case 4
            getBallPos=0;
            getEndPos=0;
            y = [aboveObjectPosition;closeFingers];
            ballGot=1;
        case 5
            getBallPos=0;
            getEndPos=0;
            y = [readyAngles;closeFingers];
            ballGot=1;
        otherwise
            y = zeros(13,1);
            getBallPos=0;
            getEndPos=0;
            ballGot=0;
    end
    
    if state == 0 && min(errorVals) >= -0.01 && max(errorVals) <=0.01
        getBallPos=1;
        stateOut = 1;
        tic;
    elseif state == 1 && min(errorVals) >= -0.01 && max(errorVals) <=0.01 && toc >= 4
%         getBallPos=1;
        stateOut = 2;
        tic;
    elseif state == 2  && toc >= 4
        stateOut = 3;
        tic;
    elseif state==3 && min(errorVals) >= -0.01 && max(errorVals) <=0.01 && toc >= 5
        stateOut = 4;
        tic;
    elseif state == 4 && min(errorVals) >= -0.01 && max(errorVals) <=0.01 && toc >= 10
        stateOut = 5;
        tic
    elseif state == 5 && min(errorVals) >= -0.01 && max(errorVals) <=0.01 && toc>=4
        stateOut = 5;
    else
        stateOut = double(state);
    end

elseif quadrupedInPosition == 2

    switch state
        case 5
            y = [readyAngles;closeFingers];
            getBallPos=0;
            getEndPos=0;
            ballGot=1;
        case 6
            getBallPos=0;
            getEndPos=0;
            y = [aboveEndPos;closeFingers];
            ballGot=1;
        case 7
            getBallPos=0;
            getEndPos=0;
            y = [endPos;closeFingers];
            ballGot=1;
        case 8
            getBallPos=0;
            getEndPos=0;
            y = [endPos;openFingers];
            ballGot=1;
        case 9
            getBallPos=0;
            getEndPos=0;
            y = [aboveEndPos;openFingers];
            ballGot=0;
        case 10
            getBallPos=0;
            getEndPos=0;
            y = [readyAngles;openFingers];
            ballGot=0;
        case 11
            getBallPos=0;
            getEndPos=0;
            y = [readyAngles;openFingers];
            ballGot=0;
        otherwise
            y = zeros(13,1);
            getBallPos=0;
            getEndPos=0;
            ballGot=0;
    end
    if state == 5 && min(errorVals) >= -0.01 && max(errorVals) <=0.01
        getEndPos=1;
        stateOut = 6;
        tic;
    elseif state == 6 && min(errorVals) >= -0.01 && max(errorVals) <=0.01 && toc >= 4
%         getBallPos=1;
        stateOut = 7;
        tic;
    elseif state == 7  && toc >= 4
        stateOut = 8;
        tic;
    elseif state==8 && min(errorVals) >= -0.01 && max(errorVals) <=0.01 && toc >= 5
        stateOut = 9;
        tic;
    elseif state == 9 && min(errorVals) >= -0.01 && max(errorVals) <=0.01 && toc >= 10
        stateOut = 10;
        tic
    elseif state == 10 && min(errorVals) >= -0.01 && max(errorVals) <=0.01 && toc>=4
        stateOut = 11;
    elseif state == 11 && min(errorVals) >= -0.01 && max(errorVals) <=0.01 && toc>=4
        stateOut = 11;
    else
        stateOut = double(state);
    end
else
    y = [readyAngles;openFingers];
    stateOut = 0;
    getBallPos=0;
    getEndPos=0;
    ballGot=0;
end

== matlab function block_manipulator/Manipulator1/Ball Tracking and Handling/MATLAB Function1 ==
  data: objectTransform output; x input; y input; z input; aboveObjectTransform output
function [objectTransform,aboveObjectTransform] = fcn(x,y,z)
rotTransform=[1 0 0;0 -1 0;0 0 -1];
F=rotTransform;
xline=F(1,:);
yline=F(2,:);
zline=F(3,:);
objectTransform = [ xline x;yline y;zline z+0.02;0 0 0 1];
aboveObjectTransform = [xline x;yline y;zline z+0.1;0 0 0 1];

== matlab function block_manipulator/Manipulator1/Subsystem1/Manipulator interpolator ==
  settings: updateMethod=DISCRETE
  data: desiredAngles input size=[7  1]; angleRangeOut output size=[1 14]; currentAngles input size=[7 1]; timeRangeOut output size=[1 14]; time input; debug output
function [angleRangeOut,timeRangeOut,debug]  = manipInterp(desiredAngles,currentAngles,time)

persistent beginState
persistent ready1
persistent ready2
persistent ready3
persistent ready4
persistent ready5
persistent ready6
persistent ready7

% persistent interval
persistent startTime
persistent angleRange
persistent timeRange

if isempty(beginState)
    beginState=transpose(currentAngles);
end

% if isempty(interval)
%     interval=0.01;
% end
if isempty(startTime)
    startTime=10;
end
if isempty(angleRange)
    angleRange=[transpose(currentAngles),transpose(currentAngles)];
end
if isempty(timeRange)
    timeRange=[ones(1,7)*0,ones(1,7)*600];
end
if isempty(ready1)
    ready1=0;
end
if isempty(ready2)
    ready2=0;
end
if isempty(ready3)
    ready3=0;
end
if isempty(ready4)
    ready4=0;
end
if isempty(ready5)
    ready5=0;
end
if isempty(ready6)
    ready6=0;
end
if isempty(ready7)
    ready7=0;
end

%timeSteps=0.01;
transferTime=3;
%calcTime=timeSteps/transferTime;
angleDif=transpose(abs(desiredAngles-currentAngles));
threshold=0.01;
TcurrentAngles=transpose(currentAngles);
if angleDif(1)>=threshold||angleDif(2)>=threshold||angleDif(3)>=threshold||angleDif(4)>=threshold||angleDif(5)>=threshold||angleDif(6)>=threshold||angleDif(7)>=threshold
    if ready1==0&&ready2==0&&ready3==0&&ready4==0&&ready5==0&&ready6==0&&ready7==0
        beginState=transpose(currentAngles);
        %interval=((desiredAngles-beginState)./calcTime);
        startTime=time;
        ready1=1;
        ready2=1;
        ready3=1;
        ready4=1;
        ready5=1;
        ready6=1;
        ready7=1;
        endTime=transferTime+startTime;
        timeRange=[ones(1,7)*startTime,ones(1,7)*endTime];
        angleRange=[beginState,transpose(desiredAngles)];
    end       
end

if angleDif(1)<=threshold
    ready1=0;
    timeRange(1)=0;
    timeRange(8)=600;
    angleRange(1)=TcurrentAngles(1);
    angleRange(8)=TcurrentAngles(1);
end
if angleDif(2)<=threshold
    ready2=0;
    timeRange(2)=0;
    timeRange(9)=600;
    angleRange(2)=TcurrentAngles(2);
    angleRange(9)=TcurrentAngles(2);
end
if angleDif(3)<=threshold
    ready3=0;
    timeRange(3)=0;
    timeRange(10)=600;
    angleRange(3)=TcurrentAngles(3);
    angleRange(10)=TcurrentAngles(3);
end
if angleDif(4)<=threshold
    ready4=0;
    timeRange(4)=0;
    timeRange(11)=600;
    angleRange(4)=TcurrentAngles(4);
    angleRange(11)=TcurrentAngles(4);
end
if angleDif(5)<=threshold
    ready5=0;
    timeRange(5)=0;
    timeRange(12)=600;
    angleRange(5)=TcurrentAngles(5);
    angleRange(12)=TcurrentAngles(5);
end
if angleDif(6)<=threshold
    ready6=0;
    timeRange(6)=0;
    timeRange(13)=600;
    angleRange(6)=TcurrentAngles(6);
    angleRange(13)=TcurrentAngles(6);
end
if angleDif(7)<=threshold
    ready7=0;
    timeRange(7)=0;
    timeRange(14)=600;
    angleRange(7)=TcurrentAngles(7);
    angleRange(14)=TcurrentAngles(7);
end

angleRangeOut=angleRange;
timeRangeOut=timeRange;
debug=angleDif;

== matlab function block_manipulator/Block controller subsystem/MATLAB Function ==
  settings: updateMethod=DISCRETE
  data: forwardVelocity output; angVelocity output; target1 input; target2 input; xpos input; ypos input; anglePos input; stopSim output; debug output
function [forwardVelocity,angVelocity,stopSim,debug] = pathChaser(target1,target2,xpos,ypos,anglePos)


%used to keep track of the current target
persistent currentTarget;
persistent path;

if isempty(currentTarget)
    currentTarget = 1;
end

if isempty(path)
    path =1;
end





rotMoveSpeed=1;
if path==1
    target=target1;
elseif path==2
    target=target2;
else
    target=target1;
end

%finds the number of targets
numTargets=size(target,1);
%sets the variable that stops the simulation to 0
stopSim=0;
%gets the x and y positions of the current target
targetx=target(currentTarget,1);
targety=target(currentTarget,2);

%finds the distance between the body of the robot and the target centre
xDiff=targetx-xpos;
yDiff=targety-ypos;
%finds the angle between the x axis of the simulation and the line pointing
%towards the target centre
targetAngle=atan2(yDiff,xDiff);

%finds the angle between the x axis of the robot and the line pointing
%toward the target centre
angDiff=targetAngle-anglePos;

%checkis if the robot has reached the final target
if currentTarget==numTargets
    if path==1
        forwardVelocity=0;
        angVelocity=0;
        pause(5);
        currentTarget=1;
        path=2;
    elseif path==2
        stopSim=1;
        forwardVelocity=0;
        angVelocity=0;
    else
       forwardVelocity=0;
        angVelocity=0; 
    end

%if not runs the path follower
else 
    %if the robot is not within 0.1m of the target
    if abs(xDiff+yDiff)>=0.1
        %if the angle between the x axis of the robot and the target is not
        %less than ~6 degrees
        if abs(angDiff)>=0.05
            %if the angle difference is positive
            if angDiff>0
                %stop and rotate left
                angVelocity=rotMoveSpeed;
                forwardVelocity=0;
            else
                %else stop and rotate right
                angVelocity=-rotMoveSpeed;
                forwardVelocity=0;
            end
        else
            %if angle is less than ~6 degrees move forward
            angVelocity=0;
            forwardVelocity=1;
        end

    else
        %if robot is within 0.1m of target check target off and set new
        %target
        currentTarget=currentTarget+1;
        forwardVelocity=0;
        angVelocity=0;
    end
end
debug=currentTarget;

== stateflow chart block_manipulator/Controller/High Level Mode Stateflow ==
  state ManipTask
    ManipTask=1;
  note: 0.35
  note: 1
  state ResetPos
    mode=0;
    forwardVelocity=0;
    angVelocity=0;
    bodyMode=1;
  state Stationary
    mode=0;
    forwardVelocity=0;
    angVelocity=0;
    bodyMode=1;
  state Turning_Right
    mode=2;
    angVelocity=rotMoveSpeed;
    forwardVelocity=0;
  state Walking
    bodyMode=0;
    mode=1;
    forwardVelocity=forwardSpeed;
    angVelocity=0;
  state Turning_Left
    mode=3;
    angVelocity=-rotMoveSpeed;
    forwardVelocity=0;
  ResetPos -> ManipTask : [stopped]
  ManipTask -> Stationary : [resetPos==0]
  Turning_Right -> ResetPos [order 2] : [resetPos==1]{pos_index=pos_index+2;bodyMode=1}
  Stationary -> ResetPos [order 2] : [resetPos==1]{pos_index=pos_index+2;bodyMode=1}
  Turning_Left -> ResetPos [order 2] : [resetPos==1]{pos_index=pos_index+2;bodyMode=1}
  Walking -> ResetPos [order 4] : [resetPos==1]{pos_index=pos_index+2;bodyMode=1}
  Stationary -> Stationary [order 3] : [target_reached]
      | {pos_index = pos_index + 1}
  (default) -> Stationary : {pos_index =2;bodyMode=0}
  Turning_Left -> Stationary [order 1] : [delta_theta < ang_threshold]
  Turning_Right -> Stationary [order 1] : [delta_theta > -ang_threshold]
  Stationary -> Walking [order 1] : [~target_reached]
  Walking -> Stationary [order 3] : [target_reached]
      | {pos_index = pos_index + 1}
  Walking -> Turning_Right [order 2] : [delta_theta < -ang_threshold]
  Walking -> Turning_Left [order 1] : [delta_theta > ang_threshold]
  data: pos_index output =0; mode output =0; target_reached input; delta_theta input; ang_threshold local =0.2; resetPos input; ManipTask output; manipState input; forwardSpeed constant double =0.5; rotMoveSpeed constant double =0.2; angVelocity output; forwardVelocity output; stopped input; bodyMode output
